simulink model "oiac_implimintation_test"  (R2024a)
settings: Solver=FixedStepAuto  StartTime=0.0  StopTime=inf  RelTol=1e-3  EnableMultiTasking=on
values from neighbouring files (symbols this model uses):
  a = 500    [InitVariables.m]
  b = 0.004    [InitVariables.m]
  Beta = 0.005    [InitVariables.m]
undefined symbols (not defined in the file or in its folder): ax, ay, az, Earth, Payload, SampleTime, vx, vy, vz, WGS84, x, y, z
libraries: px4Sensorslib x5, px4uORBlib x2, simulink x1, aerolibtransform2 x1, uavmavlinklib x1, px4lib x1
settings Model: ExtModeTrigDuration=10  Creator=zaina  LastModifiedBy=zaina
settings SolverCC: AlgebraicLoopSolver=TrustRegion  PositivePriorityOrder=on  AutoInsertRateTranBlk=on  MaxZcPerStep=1
settings OptimizationCC: EnhancedBackFolding=on  PassReuseOutputArgsAs=Individual arguments  ZeroExternalMemoryAtStartup=off  ZeroInternalMemoryAtStartup=off  MaxStackSize=64  OptimizeBlockOrder=speed  DifferentSizesBufferReuse=on  OptimizationCustomize=off  EfficientTunableParamExpr=on
settings DebuggingCC: ParameterTunabilityLossMsg=error  UnconnectedInputMsg=warning  UnconnectedOutputMsg=warning  UnconnectedLineMsg=warning  SymbolicDimsDataTypeCodeGenerationDiagnostic=none
settings HardwareCC: ProdBitPerPointer=32  ProdBitPerSizeT=32  ProdBitPerPtrDiffT=32  ProdLargestAtomicInteger=Long  ProdLargestAtomicFloat=Double  ProdWordSize=32  ProdLongLongMode=on  ProdHWDeviceType=ARM Compatible->ARM Cortex
settings ModelReferenceCC: EnableRefExpFcnMdlSchedulingChecks=on
settings SFSimCC: MATLABDynamicMemAlloc=off  SimTargetLang=C++
settings RTWCC: Description=Embedded Coder  SystemTargetFile=ert.tlc  HardwareBoard=PX4 Pixhawk 4  TLCOptions="-aInlineSetEventsForThisBaseRateFcn=TLC_FALSE -aSuppressMultiTaskScheduler=TLC_FALSE  -aRateBasedStepFcn=0"  TemplateMakefile=ert_default_tmf  Toolchain=GNU Tools for PX4 Autopilots  IncludeHyperlinkInReport=on  TargetLang=C++  GPUComputeCapability=3.5  DLArmComputeVersion=19.05
settings CodeAppCC: ForceParamTrailComments=on  IgnoreCustomStorageClasses=off  OperatorAnnotations=on  SimulinkDataObjDesc=on  SFDataObjDesc=on  InsertBlockDesc=on
settings ERTTargetCC: ExtModeTransport=3  ExtModeStaticAlloc=on  ExtModeStaticAllocSize=1024  ExtModeMexFile=ext_xcp  ExtModeIntrfLevel=Level2 - Open

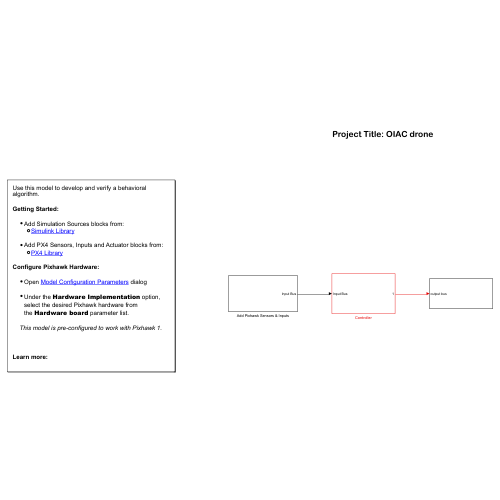
[thumbnail: Simulink's stored preview of the top-level diagram]
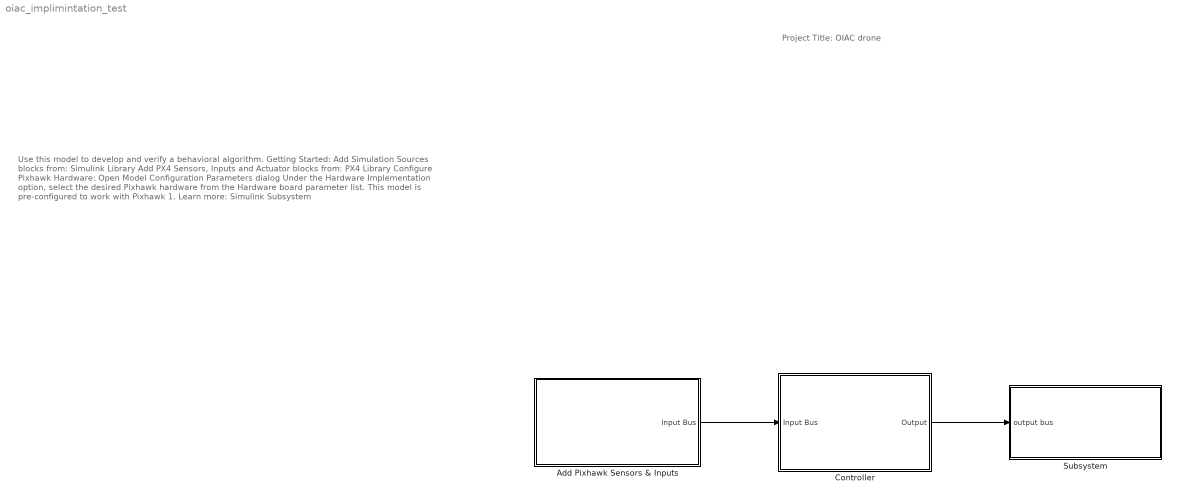
== system oiac_implimintation_test ==
  note: Project Title: OIAC drone
  note: Use this model to develop and verify a behavioral algorithm.
      |
      | Getting Started:
      |
      | Add Simulation Sources blocks from:
      | Simulink Library
      |
      | Add PX4 Sensors, Inputs and Actuator blocks from:
      | PX4 Library
      |
      | Configure Pixhawk Hardware:
      |
      | Open Model Configuration Parameters dialog
      |
      | Under the Hardware Implementation option, select the desired Pixhawk hardware from the Hardware board parameter list.
      |
      | This model is pre-configured to work with Pixhawk 1.
      |
      | Learn more:
      |
      | Simulink Subsystem
  Add Pixhawk Sensors & Inputs : Subsystem
  Controller : Subsystem
  Subsystem : Subsystem
  wires:
  Add Pixhawk Sensors & Inputs/1(Input Bus) -> Controller/1(Input Bus)
  Controller/1(Output) -> Subsystem/1(output bus)

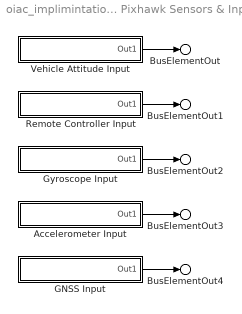
== system oiac_implimintation_test/Add Pixhawk Sensors & Inputs ==
  Accelerometer Input : Subsystem
  GNSS Input : Subsystem
  Gyroscope Input : Subsystem
  Remote Controller Input : Subsystem
  Vehicle Attitude Input : Subsystem
  BusElementOut : Outport  PortName=Input Bus  Element=Attitude
  BusElementOut1 : Outport  PortName=Input Bus  Element=RC
  BusElementOut2 : Outport  PortName=Input Bus  Element=Gyro
  BusElementOut3 : Outport  PortName=Input Bus  Element=Accelerometer
  BusElementOut4 : Outport  PortName=Input Bus  Element=GPS
  wires:
  Vehicle Attitude Input/1(Out1) -> BusElementOut/1
  Remote Controller Input/1(Out1) -> BusElementOut1/1
  GNSS Input/1(Out1) -> BusElementOut4/1
  Accelerometer Input/1(Out1) -> BusElementOut3/1
  Gyroscope Input/1(Out1) -> BusElementOut2/1

== system oiac_implimintation_test/Controller ==
  note: PX4 Attitude Control
  Input Bus : Inport  OutDataTypeStr=Bus: InputBusObject
  ARMINGControl : Subsystem
  AttitudeControl : Subsystem
  Bus Creator : BusCreator  Inputs=3  OutDataTypeStr=Bus: OutputBusObject  NonVirtualBus=on
      settings: InheritFromInputs=off
  InputConditioning : Subsystem
  failsafe : Constant  Value=0  OutDataTypeStr=boolean
  Output : Outport
  wires:
  AttitudeControl/1(Out1) -> Bus Creator/3
  failsafe/1 -> Bus Creator/2
  Input Bus/1 -> AttitudeControl/1(Input Bus), InputConditioning/1(Input Bus), ARMINGControl/1(Input Bus)
  InputConditioning/1(Normalized RC Bus) -> AttitudeControl/2(Nomralized RC bus)
  ARMINGControl/1(Out1) -> Bus Creator/1
  Bus Creator/1 -> Output/1

== system oiac_implimintation_test/Subsystem ==
  In Bus Element : Inport  PortName=output bus  Element=Arm
  In Bus Element1 : Inport  PortName=output bus  Element=Failsafe
  In Bus Element2 : Inport  PortName=output bus  Element=MotorSpeeds
  Demux : Demux
  PX4 PWM Output : px4lib/PX4 PWM Output  pwmDevice=Main  pwmChannel1_=on  pwmChannel2_=on  pwmChannel3_=on  pwmChannel4_=on  pwmChannel5_=off  pwmChannel6_=off  pwmChannel7_=off  pwmChannel8_=off
  wires:
  In Bus Element1/1 -> PX4 PWM Output/2
  In Bus Element/1 -> PX4 PWM Output/1
  In Bus Element2/1 -> Demux/1
  Demux/3 -> PX4 PWM Output/5
  Demux/1 -> PX4 PWM Output/3
  Demux/2 -> PX4 PWM Output/4
  Demux/4 -> PX4 PWM Output/6

== system oiac_implimintation_test/Add Pixhawk Sensors & Inputs/Accelerometer Input ==
  Accelerometer : px4Sensorslib/Accelerometer  uorbTimeStamp=off  BlockingMode=off  BlockTimeout=1e-3  sampleTime=1/250
  BusElementOut : Outport  PortName=Out1  Element=Accelerometer_Status
  BusElementOut1 : Outport  PortName=Out1  Element=Accelerometer_X
  BusElementOut2 : Outport  PortName=Out1  Element=Accelerometer_Y
  BusElementOut3 : Outport  PortName=Out1  Element=Accelerometer_Z
  wires:
  Accelerometer/1 -> BusElementOut/1
  Accelerometer/2 -> BusElementOut1/1
  Accelerometer/4 -> BusElementOut3/1
  Accelerometer/3 -> BusElementOut2/1

== system oiac_implimintation_test/Add Pixhawk Sensors & Inputs/GNSS Input ==
  GPS : px4Sensorslib/GPS  lat=on  lon=on  alt=on  velocity=off  course=off  gpsfix=off  numsat=off  timestamp_utc=off  BlockingMode=off  BlockTimeout=1e-3  dop=off  vel_ned=off  alt_ellipsoid=off  jamm_ind=off  timestamp=off  sampleTime=1/250
  BusElementOut : Outport  PortName=Out1  Element=GPS_Status
  BusElementOut1 : Outport  PortName=Out1  Element=Latitude
  BusElementOut2 : Outport  PortName=Out1  Element=Longitude
  BusElementOut3 : Outport  PortName=Out1  Element=Altitude
  wires:
  GPS/1 -> BusElementOut/1
  GPS/2 -> BusElementOut1/1
  GPS/3 -> BusElementOut2/1
  GPS/4 -> BusElementOut3/1

== system oiac_implimintation_test/Add Pixhawk Sensors & Inputs/Gyroscope Input ==
  Gyroscope : px4Sensorslib/Gyroscope  uorbTimeStamp=off  BlockingMode=off  BlockTimeout=1e-3  sampleTime=1/250
  BusElementOut : Outport  PortName=Out1  Element=Gyro_status
  BusElementOut1 : Outport  PortName=Out1  Element=Gyro_X
  BusElementOut2 : Outport  PortName=Out1  Element=Gyro_Y
  BusElementOut3 : Outport  PortName=Out1  Element=Gyro_Z
  wires:
  Gyroscope/1 -> BusElementOut/1
  Gyroscope/3 -> BusElementOut2/1
  Gyroscope/2 -> BusElementOut1/1
  Gyroscope/4 -> BusElementOut3/1

== system oiac_implimintation_test/Add Pixhawk Sensors & Inputs/Remote Controller Input ==
  Radio Control Transmitter : px4Sensorslib/Radio Control Transmitter  channel1=on  channel2=on  channel3=on  channel4=on  channel5=off  channel6=off  channel7=off  channel8=on  channel_count=off  rssi=off  rc_input_source=off  timestamp_last_signal=off  time_stamp=off  sampleTime=1/250  BlockingMode=off  BlockTimeout=5
  BusElementOut : Outport  PortName=Out1  Element=RC_Status
  BusElementOut1 : Outport  PortName=Out1  Element=Throttle
  BusElementOut2 : Outport  PortName=Out1  Element=Desired_Roll
  BusElementOut3 : Outport  PortName=Out1  Element=Desired_Pitch
  BusElementOut4 : Outport  PortName=Out1  Element=Desired_Yaw
  BusElementOut5 : Outport  PortName=Out1  Element=RC_Arming
  wires:
  Radio Control Transmitter/6 -> BusElementOut5/1
  Radio Control Transmitter/5 -> BusElementOut4/1
  Radio Control Transmitter/4 -> BusElementOut3/1
  Radio Control Transmitter/1 -> BusElementOut/1
  Radio Control Transmitter/3 -> BusElementOut2/1
  Radio Control Transmitter/2 -> BusElementOut1/1

== system oiac_implimintation_test/Add Pixhawk Sensors & Inputs/Vehicle Attitude Input ==
  Vehicle Attitude : px4Sensorslib/Vehicle Attitude  rollRate=off  pitchRate=off  yawRate=off  quaternion=on  uorbTimeStamp=off  BlockingMode=off  BlockTimeout=0.001  sampleTime=1/250
  BusElementOut : Outport  PortName=Out1  Element=Attitude_Status
  BusElementOut1 : Outport  PortName=Out1  Element=Attitude_Quaternions
  wires:
  Vehicle Attitude/1 -> BusElementOut/1
  Vehicle Attitude/2 -> BusElementOut1/1

== system oiac_implimintation_test/Controller/ARMINGControl ==
  In Bus Element : Inport  PortName=Input Bus  Element=RC.RC_Arming
  Compare To Constant3 : simulink/Logic and Bit Operations/Compare To Constant  relop=>=  const=uint16(1500)  OutDataTypeStr=boolean
  Out1 : Outport  VectorParamsAs1DForOutWhenUnconnected=off
  wires:
  Compare To Constant3/1 -> Out1/1
  In Bus Element/1 -> Compare To Constant3/1

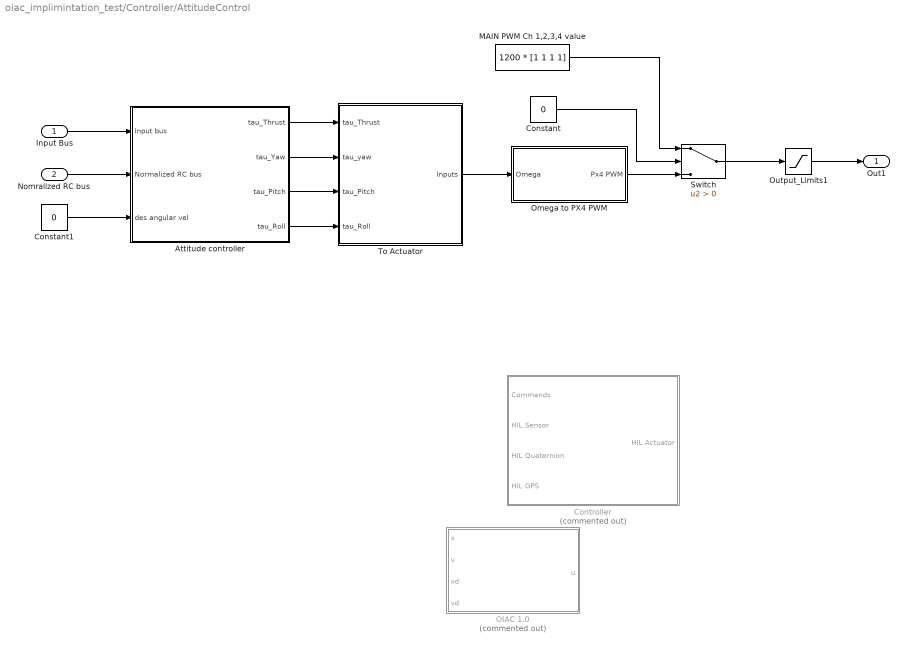
== system oiac_implimintation_test/Controller/AttitudeControl ==
  Input Bus : Inport
  Nomralized RC bus : Inport  Port=2
  Attitude controller : Subsystem
  Constant : Constant  Value=0
  Constant1 : Constant  Value=0
  "Controller " : Subsystem  Commented=on
  MAIN PWM Ch 1,2,3,4 value : Constant  Value=1200 * [1 1 1 1]  OutDataTypeStr=uint16  SampleTime=1/250
  OIAC 1.0 : Subsystem  Commented=on
  Omega to PX4 PWM : Subsystem
  Output_Limits1 : Saturate  UpperLimit=2000  LowerLimit=500
  Switch : Switch  Criteria=u2 > Threshold  SaturateOnIntegerOverflow=off  InputSameDT=off
  To Actuator : Subsystem
  Out1 : Outport
  wires:
  To Actuator/1(Inputs) -> Omega to PX4 PWM/1(Omega)
  Omega to PX4 PWM/1(Px4 PWM) -> Switch/3
  MAIN PWM Ch 1,2,3,4 value/1 -> Switch/1
  Switch/1 -> Output_Limits1/1
  Constant/1 -> Switch/2
  Attitude controller/2(tau_Yaw) -> To Actuator/2(tau_yaw)
  Attitude controller/3(tau_Pitch) -> To Actuator/3(tau_Pitch)
  Attitude controller/4(tau_Roll) -> To Actuator/4(tau_Roll)
  Constant1/1 -> Attitude controller/3(des angular vel)
  Output_Limits1/1 -> Out1/1
  Input Bus/1 -> Attitude controller/1(Input bus)
  Nomralized RC bus/1 -> Attitude controller/2(Normalized RC bus)
  Attitude controller/1(tau_Thrust) -> To Actuator/1(tau_Thrust)

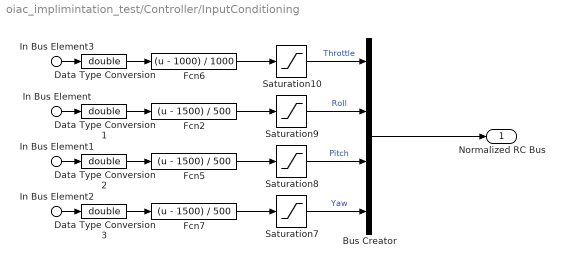
== system oiac_implimintation_test/Controller/InputConditioning ==
  In Bus Element : Inport  PortName=Input Bus  Element=RC.Desired_Roll
  In Bus Element1 : Inport  PortName=Input Bus  Element=RC.Desired_Pitch
  In Bus Element2 : Inport  PortName=Input Bus  Element=RC.Desired_Yaw
  In Bus Element3 : Inport  PortName=Input Bus  Element=RC.Throttle
  Bus Creator : BusCreator  Inputs=4  OutDataTypeStr=Bus: NormalizedRCBus
      settings: InheritFromInputs=off
  Data Type Conversion{,1..3} (4 alike) : DataTypeConversion  OutDataTypeStr=double  SaturateOnIntegerOverflow=off  RndMeth=Floor
  Fcn2 : Fcn  Expr=(u - 1500) / 500
  Fcn5 : Fcn  Expr=(u - 1500) / 500
  Fcn6 : Fcn  Expr=(u - 1000) / 1000
  Fcn7 : Fcn  Expr=(u - 1500) / 500
  Saturation10 : Saturate  UpperLimit=1  LowerLimit=0
  Saturation7 : Saturate  UpperLimit=1  LowerLimit=-1
  Saturation8 : Saturate  UpperLimit=1  LowerLimit=-1
  Saturation9 : Saturate  UpperLimit=1  LowerLimit=-1
  Normalized RC Bus : Outport
  wires:
  In Bus Element3/1 -> Data Type Conversion/1
  In Bus Element/1 -> Data Type Conversion1/1
  In Bus Element1/1 -> Data Type Conversion2/1
  Fcn7/1 -> Saturation7/1
  Fcn5/1 -> Saturation8/1
  Fcn2/1 -> Saturation9/1
  In Bus Element2/1 -> Data Type Conversion3/1
  Fcn6/1 -> Saturation10/1
  Bus Creator/1 -> Normalized RC Bus/1
  Saturation7/1 -> Bus Creator/4  "Yaw"
  Saturation8/1 -> Bus Creator/3  "Pitch"
  Saturation9/1 -> Bus Creator/2  "Roll"
  Saturation10/1 -> Bus Creator/1  "Throttle"
  Data Type Conversion/1 -> Fcn6/1
  Data Type Conversion1/1 -> Fcn2/1
  Data Type Conversion2/1 -> Fcn5/1
  Data Type Conversion3/1 -> Fcn7/1

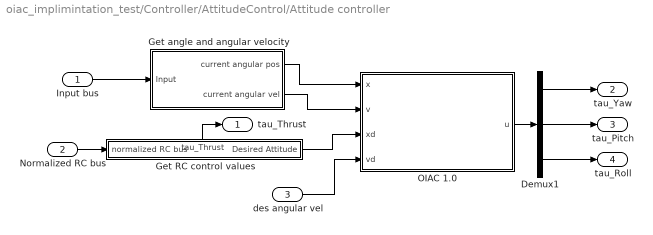
== system oiac_implimintation_test/Controller/AttitudeControl/Attitude controller ==
  Input bus : Inport
  Normalized RC bus : Inport  Port=2
  des angular vel : Inport  Port=3
  Demux1 : Demux  Outputs=3
  Get RC control values : Subsystem
      settings: PortSchema="{\"entries\":[{\"content\":{\"sides\":[{\"content\":{\"connectorIds\":[\"In1\"]},\"type\":\"ConnectorPlacement.EquallySpacedRectSide\",\"uuid\":\"d4f2e642-f139-4afb-8b32-1aebe4549dbe\"},{\"content\":{\"connectorIds\":[\"Out1\"],\"side\":\"RIGHT\"},\"type\":\"ConnectorPlacement.EquallySpacedRectSide\",\"uuid\":\"0ee46758-dfc7-4a62-8fbd-59cb0eb01f75\"},{\"content\":{\"connectorIds\":[\"Out2\"],\"side\":\"TOP\"},\"type\":\"ConnectorPlacement.EquallySpacedRectSide\",\"uuid\":\"97c85156-eef5-4db9-a7e2-7c3008b526ed\"},{\"content\":{\"side\":\"BOTTOM\"},\"type\":\"ConnectorPlacement.EquallySpacedRectSide\",\"uuid\":\"9c2d9dad-2c34-460b-8d31-41aca7aeb9a1\"}]},\"type\":\"ConnectorPlacement.EquallySpacedConnector\",\"uuid\":\"3a83a1b3-2f36-4168-b552-4bb8228b6c94\"}],\"packageUris\":[\"http://schema.mathworks.com/mf0/Connector/R2020b\"],\"version\":\"1.0\"}"
  Get angle and angular velocity : Subsystem
  OIAC 1.0 : Subsystem
  tau_Thrust : Outport
  tau_Yaw : Outport  Port=2
  tau_Pitch : Outport  Port=3
  tau_Roll : Outport  Port=4
  wires:
  Get RC control values/1(Desired Attitude) -> OIAC 1.0/3(xd)
  Input bus/1 -> Get angle and angular velocity/1(Input)
  Normalized RC bus/1 -> Get RC control values/1(normalized RC bus)
  Get angle and angular velocity/1(current angular pos) -> OIAC 1.0/1(x)
  Demux1/2 -> tau_Pitch/1
  des angular vel/1 -> OIAC 1.0/4(vd)
  Get angle and angular velocity/2(current angular vel) -> OIAC 1.0/2(v)
  OIAC 1.0/1(u) -> Demux1/1
  Demux1/1 -> tau_Yaw/1
  Demux1/3 -> tau_Roll/1
  Get RC control values/2(tau_Thrust) -> tau_Thrust/1

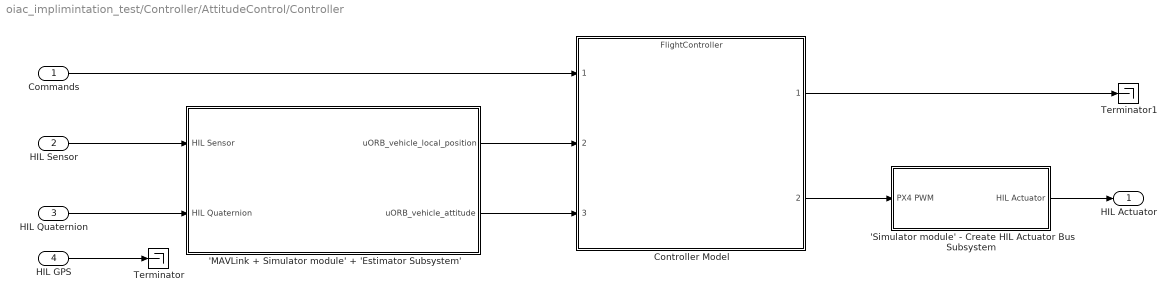
== system oiac_implimintation_test/Controller/AttitudeControl/Controller  ==
  Commands : Inport
  HIL Sensor : Inport  Port=2
  HIL Quaternion : Inport  Port=3
  HIL GPS : Inport  Port=4
  'MAVLink + Simulator module' + 'Estimator Subsystem' : Subsystem
      settings: PortSchema="{\"entries\":[{\"content\":{\"sides\":[{\"content\":{\"connectorIds\":[]},\"type\":\"ConnectorPlacement.EquallySpacedRectSide\",\"uuid\":\"18f19b7f-7de0-4ac4-a24f-d8ceb747f924\"},{\"content\":{\"connectorIds\":[],\"side\":\"RIGHT\"},\"type\":\"ConnectorPlacement.EquallySpacedRectSide\",\"uuid\":\"b474fbae-f8e2-4c2b-be96-a63ee47992dd\"},{\"content\":{\"connectorIds\":[\"In1\",\"In2\"],\"side\":\"TOP\"},\"type\":\"ConnectorPlacement.EquallySpacedRectSide\",\"uuid\":\"67540526-de5d-4152-a323-fd05419e6390\"},{\"content\":{\"connectorIds\":[\"Out1\",\"Out2\"],\"side\":\"BOTTOM\"},\"type\":\"ConnectorPlacement.EquallySpacedRectSide\",\"uuid\":\"c51ef1bd-db79-4835-87f1-e9dccd8fce9f\"},{\"content\":{\"connectorIds\":[],\"side\":\"HIDDEN\"},\"type\":\"ConnectorPlacement.EquallySpacedRectSide\",\"uuid\":\"82a3913e-38ee-407a-aef4-9df458d840d7\"}]},\"type\":\"ConnectorPlacement.EquallySpacedConnector\",\"uuid\":\"5015a705-00cf-433b-8716-d3e1ebe8eda0\"}],\"packageUris\":[\"http://schema.mathworks.com/mf0/Connector/R2020b\"],\"version\":\"1.0\"}"
  'Simulator module' - Create HIL Actuator Bus Subsystem : Subsystem
  Controller Model : ModelReference  ModelNameDialog=FlightController.slx  SimulationMode=Normal  ModelReferenceVersion=8.0
  Terminator : Terminator
  Terminator1 : Terminator
  HIL Actuator : Outport
  wires:
  Controller Model/2 -> 'Simulator module' - Create HIL Actuator Bus Subsystem/1(PX4 PWM)
  'Simulator module' - Create HIL Actuator Bus Subsystem/1(HIL Actuator) -> HIL Actuator/1
  HIL Sensor/1 -> 'MAVLink + Simulator module' + 'Estimator Subsystem'/2(HIL Sensor)
  HIL Quaternion/1 -> 'MAVLink + Simulator module' + 'Estimator Subsystem'/1(HIL Quaternion)
  Commands/1 -> Controller Model/1
  'MAVLink + Simulator module' + 'Estimator Subsystem'/2(uORB_vehicle_local_position) -> Controller Model/2
  'MAVLink + Simulator module' + 'Estimator Subsystem'/1(uORB_vehicle_attitude) -> Controller Model/3
  HIL GPS/1 -> Terminator/1
  Controller Model/1 -> Terminator1/1

== system oiac_implimintation_test/Controller/AttitudeControl/OIAC 1.0 ==
  x : Inport
  v : Inport  Port=2
  xd : Inport  Port=3
  vd : Inport  Port=4
  Subsystem : Subsystem
  Subsystem2 : Subsystem
  u : Outport
  wires:
  vd/1 -> Subsystem/4(vd)
  v/1 -> Subsystem/3(v)
  Subsystem2/1(u) -> u/1
  Subsystem/1(e) -> Subsystem2/1(e)
  Subsystem/2(e_dot) -> Subsystem2/2(edot)
  x/1 -> Subsystem/1(x)
  xd/1 -> Subsystem/2(xd)

== system oiac_implimintation_test/Controller/AttitudeControl/Omega to PX4 PWM ==
  Omega : Inport
  Constant : Constant  Value=500  SampleTime=-1
  Data Type Conversion : DataTypeConversion  OutDataTypeStr=uint16  SaturateOnIntegerOverflow=off  RndMeth=Floor
  Gain : Gain  Gain=1500
  Sum : Sum  Inputs=|++
  Px4 PWM : Outport
  wires:
  Data Type Conversion/1 -> Px4 PWM/1
  Sum/1 -> Data Type Conversion/1
  Omega/1 -> Gain/1
  Constant/1 -> Sum/2
  Gain/1 -> Sum/1

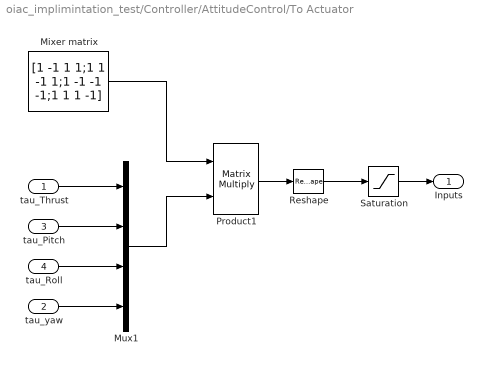
== system oiac_implimintation_test/Controller/AttitudeControl/To Actuator ==
  tau_Thrust : Inport
  tau_yaw : Inport  Port=2
  tau_Pitch : Inport  Port=3
  tau_Roll : Inport  Port=4
  Mixer matrix : Constant  Value=[1 -1 1 1;1 1 -1 1;1 -1 -1 -1;1 1 1 -1]  OutDataTypeStr=Inherit: Inherit via back propagation
  Mux1 : Mux
  Product1 : Product  Multiplication=Matrix(*)  RndMeth=Zero
  Reshape : Reshape  OutputDimensionality=Row vector (2-D)
  Saturation : Saturate  UpperLimit=1  LowerLimit=0
  Inputs : Outport
  wires:
  Mixer matrix/1 -> Product1/1
  Mux1/1 -> Product1/2
  tau_Thrust/1 -> Mux1/1
  Product1/1 -> Reshape/1
  Saturation/1 -> Inputs/1
  tau_Pitch/1 -> Mux1/2
  tau_Roll/1 -> Mux1/3
  tau_yaw/1 -> Mux1/4
  Reshape/1 -> Saturation/1

== system oiac_implimintation_test/Controller/AttitudeControl/Attitude controller/Get RC control values ==
  In Bus Element : Inport  PortName=normalized RC bus  Element=Roll
  In Bus Element1 : Inport  PortName=normalized RC bus  Element=Pitch
  In Bus Element2 : Inport  PortName=normalized RC bus  Element=Yaw
  BusElementIn : Inport  PortName=normalized RC bus  Element=Throttle
  Mux : Mux  Inputs=3
  Desired Attitude : Outport
  tau_Thrust : Outport  Port=2
  wires:
  In Bus Element2/1 -> Mux/3
  In Bus Element1/1 -> Mux/2
  In Bus Element/1 -> Mux/1
  Mux/1 -> Desired Attitude/1
  BusElementIn/1 -> tau_Thrust/1

== system oiac_implimintation_test/Controller/AttitudeControl/Attitude controller/Get angle and angular velocity ==
  In Bus Element : Inport  PortName=Input  Element=Attitude.Attitude_Quaternions
  In Bus Element1 : Inport  PortName=Input  Element=Gyro.Gyro_X
  In Bus Element2 : Inport  PortName=Input  Element=Gyro.Gyro_Y
  In Bus Element3 : Inport  PortName=Input  Element=Gyro.Gyro_Z
  Mux : Mux  Inputs=3
  Mux1 : Mux  Inputs=3
  quat2eul : MATLAB Function  TreatAsAtomicUnit=on
  current angular pos : Outport
  current angular vel : Outport  Port=2
  wires:
  In Bus Element3/1 -> Mux1/3
  In Bus Element2/1 -> Mux1/2
  In Bus Element/1 -> quat2eul/1(q)
  In Bus Element1/1 -> Mux1/1
  quat2eul/3(psi) -> Mux/3
  quat2eul/2(theta) -> Mux/2
  quat2eul/1(phi) -> Mux/1
  Mux1/1 -> current angular vel/1
  Mux/1 -> current angular pos/1

== system oiac_implimintation_test/Controller/AttitudeControl/Attitude controller/OIAC 1.0 ==
  x : Inport
  v : Inport  Port=2
  xd : Inport  Port=3
  vd : Inport  Port=4
  Subsystem : Subsystem
  Subsystem2 : Subsystem
  u : Outport
  wires:
  vd/1 -> Subsystem/4(vd)
  v/1 -> Subsystem/3(v)
  Subsystem2/1(u) -> u/1
  Subsystem/1(e) -> Subsystem2/1(e)
  Subsystem/2(e_dot) -> Subsystem2/2(edot)
  x/1 -> Subsystem/1(x)
  xd/1 -> Subsystem/2(xd)

== system oiac_implimintation_test/Controller/AttitudeControl/Controller /'MAVLink + Simulator module' + 'Estimator Subsystem' ==
  HIL Quaternion : Inport
  HIL Sensor : Inport  Port=2
  Vehicle Attitude : Subsystem
  Vehicle Local Position : Subsystem
  uORB_vehicle_attitude : Outport
  uORB_vehicle_local_position : Outport  Port=2
  wires:
  HIL Quaternion/1 -> Vehicle Attitude/1(HIL Quaternion), Vehicle Local Position/1(HIL_Quaternion)
  HIL Sensor/1 -> Vehicle Local Position/2(HIL_Sensor), Vehicle Attitude/2(HIL Sensor)
  Vehicle Local Position/1(uORB_vehicle_local_position) -> uORB_vehicle_local_position/1
  Vehicle Attitude/1(uORB_vehicle_attitude) -> uORB_vehicle_attitude/1

== system oiac_implimintation_test/Controller/AttitudeControl/Controller /'Simulator module' - Create HIL Actuator Bus Subsystem ==
  PX4 PWM : Inport
  Bus Assignment : BusAssignment  AssignedSignals=Payload.time_usec,Payload.flags,Payload.controls,Payload.mode
  Constant : Constant  Value=zeros(1,12)  OutDataTypeStr=Inherit: Inherit via back propagation  SampleTime=SampleTime
  Constant1 : Constant  Value=0  OutDataTypeStr=Inherit: Inherit via back propagation  SampleTime=SampleTime
  Constant2 : Constant  Value=0  OutDataTypeStr=Inherit: Inherit via back propagation  SampleTime=SampleTime
  Data Type Conversion : DataTypeConversion  SaturateOnIntegerOverflow=off  RndMeth=Floor
  MAVLink Blank Message : uavmavlinklib/MAVLink Blank Message  dialectSource=Select from standard MAVLink dialects  dialect=common.xml  dialectCustom=common.xml  version=2  messageType=HIL_ACTUATOR_CONTROLS  SystemID=1  ComponentID=1  SampleTime=SampleTime
  Mux : Mux  Inputs=2
  HIL Actuator : Outport
  wires:
  MAVLink Blank Message/1 -> Bus Assignment/1
  Bus Assignment/1 -> HIL Actuator/1
  PX4 PWM/1 -> Mux/1
  Constant/1 -> Mux/2
  Mux/1 -> Data Type Conversion/1
  Constant2/1 -> Bus Assignment/3, Bus Assignment/2
  Constant1/1 -> Bus Assignment/5
  Data Type Conversion/1 -> Bus Assignment/4

== system oiac_implimintation_test/Controller/AttitudeControl/OIAC 1.0/Subsystem ==
  x : Inport
  xd : Inport  Port=2
  v : Inport  Port=3
  vd : Inport  Port=4
  Subtract : Sum  Inputs=+-
  Subtract1 : Sum  Inputs=+-
  e : Outport
  e_dot : Outport  Port=2
  wires:
  vd/1 -> Subtract1/2
  v/1 -> Subtract1/1
  Subtract1/1 -> e_dot/1
  x/1 -> Subtract/1
  Subtract/1 -> e/1
  xd/1 -> Subtract/2

== system oiac_implimintation_test/Controller/AttitudeControl/OIAC 1.0/Subsystem2 ==
  e : Inport
  edot : Inport  Port=2
  Constant : Constant  Value=0.5
  Constant1 : Constant  Value=0.2
  Constant2 : Constant  Value=0.4
  Subsystem1 : Subsystem
  u : Outport
  wires:
  Subsystem1/1(u) -> u/1
  Constant2/1 -> Subsystem1/5(b)
  edot/1 -> Subsystem1/4(edot)
  e/1 -> Subsystem1/3(e)
  Constant/1 -> Subsystem1/2(beta)
  Constant1/1 -> Subsystem1/1(a)

== system oiac_implimintation_test/Controller/AttitudeControl/Attitude controller/OIAC 1.0/Subsystem ==
  x : Inport
  xd : Inport  Port=2
  v : Inport  Port=3
  vd : Inport  Port=4
  Subtract : Sum  Inputs=+-
  Subtract1 : Sum  Inputs=+-
  e : Outport
  e_dot : Outport  Port=2
  wires:
  vd/1 -> Subtract1/2
  v/1 -> Subtract1/1
  Subtract1/1 -> e_dot/1
  x/1 -> Subtract/1
  Subtract/1 -> e/1
  xd/1 -> Subtract/2

== system oiac_implimintation_test/Controller/AttitudeControl/Attitude controller/OIAC 1.0/Subsystem2 ==
  e : Inport
  edot : Inport  Port=2
  Constant : Constant  Value=Beta
  Constant1 : Constant  Value=a
  Constant2 : Constant  Value=b
  Subsystem1 : Subsystem
  u : Outport
  wires:
  Subsystem1/1(u) -> u/1
  Constant2/1 -> Subsystem1/5(b)
  edot/1 -> Subsystem1/4(edot)
  e/1 -> Subsystem1/3(e)
  Constant/1 -> Subsystem1/2(beta)
  Constant1/1 -> Subsystem1/1(a)

== system oiac_implimintation_test/Controller/AttitudeControl/Controller /'MAVLink + Simulator module' + 'Estimator Subsystem'/Vehicle Attitude ==
  HIL Quaternion : Inport
  HIL Sensor : Inport  Port=2
  Bus Assignment : BusAssignment  AssignedSignals=q
  Bus Selector : BusSelector  OutputSignals=Payload.attitude_quaternion
  Data Type Conversion : DataTypeConversion  SaturateOnIntegerOverflow=off  RndMeth=Floor
  PX4 uORB Message : px4uORBlib/PX4 uORB Message  uORBTopic=vehicle_attitude  SampleTime=SampleTime  selectInstance=vehicle_attitude
  Terminator : Terminator
  uORB_vehicle_attitude : Outport
  wires:
  HIL Quaternion/1 -> Bus Selector/1
  Data Type Conversion/1 -> Bus Assignment/2
  PX4 uORB Message/1 -> Bus Assignment/1
  Bus Assignment/1 -> uORB_vehicle_attitude/1
  HIL Sensor/1 -> Terminator/1
  Bus Selector/1 -> Data Type Conversion/1  "<attitude_quaternion>"

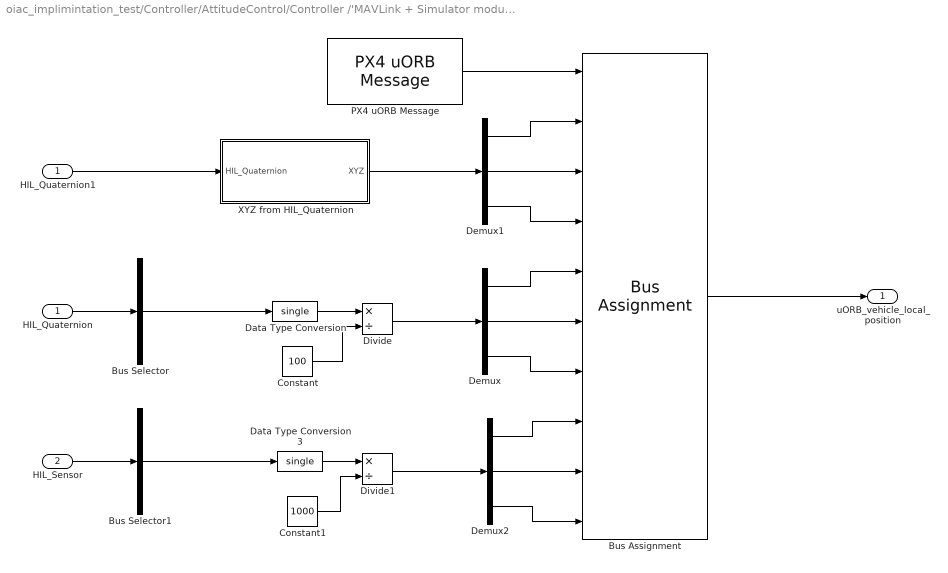
== system oiac_implimintation_test/Controller/AttitudeControl/Controller /'MAVLink + Simulator module' + 'Estimator Subsystem'/Vehicle Local Position ==
  HIL_Quaternion : Inport
  HIL_Sensor : Inport  Port=2
  Bus Assignment : BusAssignment  AssignedSignals=x,y,z,vx,vy,vz,ax,ay,az
  Bus Selector : BusSelector  OutputSignals=Payload.vx,Payload.vy,Payload.vz  OutputAsBus=on
  Bus Selector1 : BusSelector  OutputSignals=Payload.xacc,Payload.yacc,Payload.zacc  OutputAsBus=on
  Constant : Constant  Value=100  OutDataTypeStr=single  SampleTime=SampleTime
  Constant1 : Constant  Value=1000  OutDataTypeStr=single  SampleTime=SampleTime
  Data Type Conversion : DataTypeConversion  OutDataTypeStr=single  SaturateOnIntegerOverflow=off  RndMeth=Floor
  Data Type Conversion3 : DataTypeConversion  OutDataTypeStr=single  SaturateOnIntegerOverflow=off  RndMeth=Floor
  Demux : Demux  Outputs=3
  Demux1 : Demux  Outputs=3
  Demux2 : Demux  Outputs=3
  Divide : Product  Inputs=*/
  Divide1 : Product  Inputs=*/
  HIL_Quaternion1 : InportShadow
  PX4 uORB Message : px4uORBlib/PX4 uORB Message  uORBTopic=vehicle_local_position  SampleTime=SampleTime  selectInstance=vehicle_local_position
  XYZ from HIL_Quaternion : Subsystem
  uORB_vehicle_local_position : Outport
  wires:
  Bus Assignment/1 -> uORB_vehicle_local_position/1
  PX4 uORB Message/1 -> Bus Assignment/1
  Demux/3 -> Bus Assignment/7
  Bus Selector/1 -> Data Type Conversion/1
  Demux/1 -> Bus Assignment/5
  Demux/2 -> Bus Assignment/6
  Demux1/3 -> Bus Assignment/4
  Demux1/1 -> Bus Assignment/2
  Demux1/2 -> Bus Assignment/3
  Data Type Conversion/1 -> Divide/1
  HIL_Quaternion/1 -> Bus Selector/1
  Divide/1 -> Demux/1
  Constant/1 -> Divide/2
  Demux2/2 -> Bus Assignment/9
  Demux2/1 -> Bus Assignment/8
  Demux2/3 -> Bus Assignment/10
  Divide1/1 -> Demux2/1
  Bus Selector1/1 -> Data Type Conversion3/1
  HIL_Sensor/1 -> Bus Selector1/1
  Data Type Conversion3/1 -> Divide1/1
  Constant1/1 -> Divide1/2
  HIL_Quaternion1/1 -> XYZ from HIL_Quaternion/1(HIL_Quaternion)
  XYZ from HIL_Quaternion/1(XYZ) -> Demux1/1

== system oiac_implimintation_test/Controller/AttitudeControl/OIAC 1.0/Subsystem2/Subsystem1 ==
  a : Inport
  beta : Inport  Port=2
  e : Inport  Port=3
  edot : Inport  Port=4
  b : Inport  Port=5
  MATLAB Function : MATLAB Function  TreatAsAtomicUnit=on
  Subsystem2 : Subsystem
  u : Outport
  wires:
  MATLAB Function/1(u) -> u/1
  Subsystem2/2(K) -> MATLAB Function/2(K)
  Subsystem2/3(D) -> MATLAB Function/4(D)
  Subsystem2/1(F) -> MATLAB Function/1(F)
  e/1 -> MATLAB Function/3(e), Subsystem2/4(e)
  b/1 -> Subsystem2/3(b)
  edot/1 -> MATLAB Function/5(edot), Subsystem2/5(edot)
  a/1 -> Subsystem2/1(a)
  beta/1 -> Subsystem2/2(beta)

== system oiac_implimintation_test/Controller/AttitudeControl/Attitude controller/OIAC 1.0/Subsystem2/Subsystem1 ==
  a : Inport
  beta : Inport  Port=2
  e : Inport  Port=3
  edot : Inport  Port=4
  b : Inport  Port=5
  MATLAB Function : MATLAB Function  TreatAsAtomicUnit=on
  Subsystem2 : Subsystem
  u : Outport
  wires:
  MATLAB Function/1(u) -> u/1
  Subsystem2/2(K) -> MATLAB Function/2(K)
  Subsystem2/3(D) -> MATLAB Function/4(D)
  Subsystem2/1(F) -> MATLAB Function/1(F)
  e/1 -> MATLAB Function/3(e), Subsystem2/4(e)
  b/1 -> Subsystem2/3(b)
  edot/1 -> MATLAB Function/5(edot), Subsystem2/5(edot)
  a/1 -> Subsystem2/1(a)
  beta/1 -> Subsystem2/2(beta)

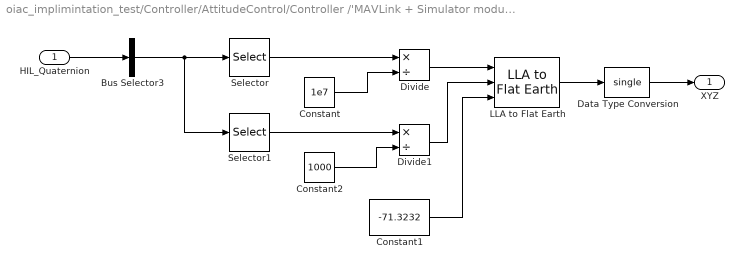
== system oiac_implimintation_test/Controller/AttitudeControl/Controller /'MAVLink + Simulator module' + 'Estimator Subsystem'/Vehicle Local Position/XYZ from HIL_Quaternion ==
  HIL_Quaternion : Inport
  Bus Selector3 : BusSelector  OutputSignals=Payload.lat,Payload.lon,Payload.alt  OutputAsBus=on
  Constant : Constant  Value=1e7  OutDataTypeStr=double
  Constant1 : Constant  Value=-71.3232  OutDataTypeStr=double
  Constant2 : Constant  Value=1000  OutDataTypeStr=double
  Data Type Conversion : DataTypeConversion  OutDataTypeStr=single  SaturateOnIntegerOverflow=off  RndMeth=Floor
  Divide : Product  Inputs=*/
  Divide1 : Product  Inputs=*/
  LLA to Flat Earth : aerolibtransform2/LLA to Flat Earth  units=Metric (MKS)  ptype=Earth (WGS84)  F=1/298.257223563  R=6378137  refPosPort=off  LL0=[0 10]  psi=0
  Selector : Selector  InputPortWidth=3  IndexOptions=Index vector (dialog)  Indices=[1:2]  OutputSizes=1
  Selector1 : Selector  InputPortWidth=3  IndexOptions=Index vector (dialog)  Indices=[3]  OutputSizes=1
  XYZ : Outport
  wires:
  HIL_Quaternion/1 -> Bus Selector3/1
  Constant1/1 -> LLA to Flat Earth/3
  Constant/1 -> Divide/2
  Bus Selector3/1 -> Selector1/1, Selector/1
  Selector/1 -> Divide/1
  Constant2/1 -> Divide1/2
  Selector1/1 -> Divide1/1
  Divide/1 -> LLA to Flat Earth/1
  Divide1/1 -> LLA to Flat Earth/2
  LLA to Flat Earth/1 -> Data Type Conversion/1
  Data Type Conversion/1 -> XYZ/1

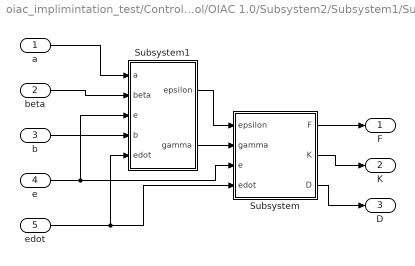
== system oiac_implimintation_test/Controller/AttitudeControl/OIAC 1.0/Subsystem2/Subsystem1/Subsystem2 ==
  a : Inport
  beta : Inport  Port=2
  b : Inport  Port=3
  e : Inport  Port=4
  edot : Inport  Port=5
  Subsystem : Subsystem
  Subsystem1 : Subsystem
  F : Outport
  K : Outport  Port=2
  D : Outport  Port=3
  wires:
  Subsystem/3(D) -> D/1
  Subsystem/2(K) -> K/1
  Subsystem/1(F) -> F/1
  edot/1 -> Subsystem1/5(edot), Subsystem/4(edot)
  Subsystem1/2(gamma) -> Subsystem/2(gamma)
  e/1 -> Subsystem1/3(e), Subsystem/3(e)
  Subsystem1/1(epsilon) -> Subsystem/1(epsilon)
  beta/1 -> Subsystem1/2(beta)
  b/1 -> Subsystem1/4(b)
  a/1 -> Subsystem1/1(a)

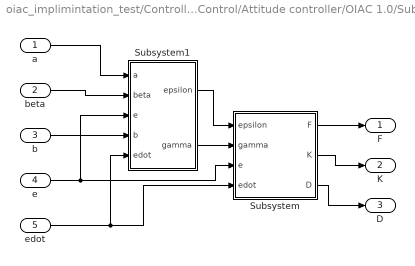
== system oiac_implimintation_test/Controller/AttitudeControl/Attitude controller/OIAC 1.0/Subsystem2/Subsystem1/Subsystem2 ==
  a : Inport
  beta : Inport  Port=2
  b : Inport  Port=3
  e : Inport  Port=4
  edot : Inport  Port=5
  Subsystem : Subsystem
  Subsystem1 : Subsystem
  F : Outport
  K : Outport  Port=2
  D : Outport  Port=3
  wires:
  Subsystem/3(D) -> D/1
  Subsystem/2(K) -> K/1
  Subsystem/1(F) -> F/1
  edot/1 -> Subsystem1/5(edot), Subsystem/4(edot)
  Subsystem1/2(gamma) -> Subsystem/2(gamma)
  e/1 -> Subsystem1/3(e), Subsystem/3(e)
  Subsystem1/1(epsilon) -> Subsystem/1(epsilon)
  beta/1 -> Subsystem1/2(beta)
  b/1 -> Subsystem1/4(b)
  a/1 -> Subsystem1/1(a)

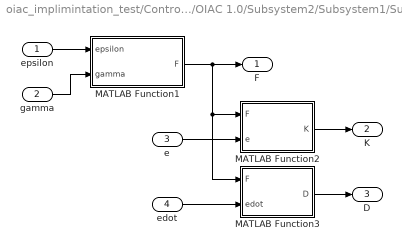
== system oiac_implimintation_test/Controller/AttitudeControl/OIAC 1.0/Subsystem2/Subsystem1/Subsystem2/Subsystem ==
  epsilon : Inport
  gamma : Inport  Port=2
  e : Inport  Port=3
  edot : Inport  Port=4
  MATLAB Function1 : MATLAB Function  TreatAsAtomicUnit=on
  MATLAB Function2 : MATLAB Function  TreatAsAtomicUnit=on
  MATLAB Function3 : MATLAB Function  TreatAsAtomicUnit=on
  F : Outport
  K : Outport  Port=2
  D : Outport  Port=3
  wires:
  MATLAB Function3/1(D) -> D/1
  MATLAB Function2/1(K) -> K/1
  MATLAB Function1/1(F) -> F/1, MATLAB Function3/1(F), MATLAB Function2/1(F)
  epsilon/1 -> MATLAB Function1/1(epsilon)
  gamma/1 -> MATLAB Function1/2(gamma)
  e/1 -> MATLAB Function2/2(e)
  edot/1 -> MATLAB Function3/2(edot)

== system oiac_implimintation_test/Controller/AttitudeControl/OIAC 1.0/Subsystem2/Subsystem1/Subsystem2/Subsystem1 ==
  a : Inport
  beta : Inport  Port=2
  e : Inport  Port=3
  b : Inport  Port=4
  edot : Inport  Port=5
  MATLAB Function4 : MATLAB Function  TreatAsAtomicUnit=on
  MATLAB Function5 : MATLAB Function  TreatAsAtomicUnit=on
  epsilon : Outport
  gamma : Outport  Port=2
  wires:
  MATLAB Function5/1(gamma) -> gamma/1
  MATLAB Function4/1(epsilon) -> MATLAB Function5/3(epsilon), epsilon/1
  edot/1 -> MATLAB Function4/2(edot)
  b/1 -> MATLAB Function5/2(b)
  e/1 -> MATLAB Function4/1(e)
  beta/1 -> MATLAB Function4/3(beta)
  a/1 -> MATLAB Function5/1(a)

== system oiac_implimintation_test/Controller/AttitudeControl/Attitude controller/OIAC 1.0/Subsystem2/Subsystem1/Subsystem2/Subsystem ==
  epsilon : Inport
  gamma : Inport  Port=2
  e : Inport  Port=3
  edot : Inport  Port=4
  MATLAB Function1 : MATLAB Function  TreatAsAtomicUnit=on
  MATLAB Function2 : MATLAB Function  TreatAsAtomicUnit=on
  MATLAB Function3 : MATLAB Function  TreatAsAtomicUnit=on
  F : Outport
  K : Outport  Port=2
  D : Outport  Port=3
  wires:
  MATLAB Function3/1(D) -> D/1
  MATLAB Function2/1(K) -> K/1
  MATLAB Function1/1(F) -> F/1, MATLAB Function3/1(F), MATLAB Function2/1(F)
  epsilon/1 -> MATLAB Function1/1(epsilon)
  gamma/1 -> MATLAB Function1/2(gamma)
  e/1 -> MATLAB Function2/2(e)
  edot/1 -> MATLAB Function3/2(edot)

== system oiac_implimintation_test/Controller/AttitudeControl/Attitude controller/OIAC 1.0/Subsystem2/Subsystem1/Subsystem2/Subsystem1 ==
  a : Inport
  beta : Inport  Port=2
  e : Inport  Port=3
  b : Inport  Port=4
  edot : Inport  Port=5
  MATLAB Function4 : MATLAB Function  TreatAsAtomicUnit=on
  MATLAB Function5 : MATLAB Function  TreatAsAtomicUnit=on
  epsilon : Outport
  gamma : Outport  Port=2
  wires:
  MATLAB Function5/1(gamma) -> gamma/1
  MATLAB Function4/1(epsilon) -> MATLAB Function5/3(epsilon), epsilon/1
  edot/1 -> MATLAB Function4/2(edot)
  b/1 -> MATLAB Function5/2(b)
  e/1 -> MATLAB Function4/1(e)
  beta/1 -> MATLAB Function4/3(beta)
  a/1 -> MATLAB Function5/1(a)

== matlab function oiac_implimintation_test/Controller/AttitudeControl/Attitude controller/OIAC 1.0/Subsystem2/Subsystem1/Subsystem2/Subsystem/MATLAB Function3 ==
  data: F input; D output; edot input
function D = fcn(F, edot)
D = F*edot';

== matlab function oiac_implimintation_test/Controller/AttitudeControl/Attitude controller/OIAC 1.0/Subsystem2/Subsystem1/Subsystem2/Subsystem1/MATLAB Function4 ==
  data: e input; epsilon output; edot input; beta input
function epsilon = fcn(e, edot, beta)
epsilon = e + beta*edot;

== matlab function oiac_implimintation_test/Controller/AttitudeControl/OIAC 1.0/Subsystem2/Subsystem1/MATLAB Function ==
  data: F input; u output; K input; e input; D input; edot input
function u = fcn(F, K, e, D, edot)
u = -F - K*e - D*edot;

== matlab function oiac_implimintation_test/Controller/AttitudeControl/Attitude controller/OIAC 1.0/Subsystem2/Subsystem1/Subsystem2/Subsystem1/MATLAB Function5 ==
  data: a input; gamma output; b input; epsilon input
function gamma = fcn(a, b, epsilon)
gamma = a/(1 + b*norm(epsilon)^2);

== matlab function oiac_implimintation_test/Controller/AttitudeControl/OIAC 1.0/Subsystem2/Subsystem1/Subsystem2/Subsystem/MATLAB Function1 ==
  data: epsilon input; F output; gamma input
function F = fcn(epsilon, gamma)
F = epsilon/gamma;

== matlab function oiac_implimintation_test/Controller/AttitudeControl/OIAC 1.0/Subsystem2/Subsystem1/Subsystem2/Subsystem/MATLAB Function2 ==
  data: F input; K output; e input
function K = fcn(F, e)
K = F*e';

== matlab function oiac_implimintation_test/Controller/AttitudeControl/OIAC 1.0/Subsystem2/Subsystem1/Subsystem2/Subsystem/MATLAB Function3 ==
  data: F input; D output; edot input
function D = fcn(F, edot)
D = F*edot';

== matlab function oiac_implimintation_test/Controller/AttitudeControl/OIAC 1.0/Subsystem2/Subsystem1/Subsystem2/Subsystem1/MATLAB Function4 ==
  data: e input; epsilon output; edot input; beta input
function epsilon = fcn(e, edot, beta)
epsilon = e + beta*edot;

== matlab function oiac_implimintation_test/Controller/AttitudeControl/OIAC 1.0/Subsystem2/Subsystem1/Subsystem2/Subsystem1/MATLAB Function5 ==
  data: a input; gamma output; b input; epsilon input
function gamma = fcn(a, b, epsilon)
gamma = a/(1 + b*norm(epsilon)^2);

== matlab function oiac_implimintation_test/Controller/AttitudeControl/Attitude controller/OIAC 1.0/Subsystem2/Subsystem1/MATLAB Function ==
  data: F input; u output; K input; e input; D input; edot input
function u = fcn(F, K, e, D, edot)
u = -F - K*e - D*edot;

== matlab function oiac_implimintation_test/Controller/AttitudeControl/Attitude controller/OIAC 1.0/Subsystem2/Subsystem1/Subsystem2/Subsystem/MATLAB Function1 ==
  data: epsilon input; F output; gamma input
function F = fcn(epsilon, gamma)
F = epsilon/gamma;

== matlab function oiac_implimintation_test/Controller/AttitudeControl/Attitude controller/OIAC 1.0/Subsystem2/Subsystem1/Subsystem2/Subsystem/MATLAB Function2 ==
  data: F input; K output; e input
function K = fcn(F, e)
K = F*e';

== matlab function oiac_implimintation_test/Controller/AttitudeControl/Attitude controller/Get angle and angular velocity/quat2eul ==
  data: q input; phi output; theta output; psi output
function [phi,theta,psi] = quat2eul(q)

% Quaternion conversion to Euler angles based on the PX4 Firmware v1.6.5
% release.

phi = atan2(2*(q(1)*q(2) + q(3)* q(4)), q(1)^2 - q(2)^2 - q(3)^2 + q(4)^2);
theta = asin(-2*(q(2)*q(4) - q(1)*q(3)));
psi = atan2(2*(q(2)*q(3) + q(1)* q(4)), q(1)^2 + q(2)^2 - q(3)^2 - q(4)^2);

end
